simulink model "NDT_Localization"  (R2022a)
settings: Solver=FixedStepAuto  StartTime=0.0  StopTime=10.0  RelTol=1e-3
model workspace (MAT data in the model file):
  SL_ROS_VariableLengthArrays_MaxSizes : object (value not decoded)
undefined symbols (not defined in the file or in its folder): null
libraries: ros2lib x9, robotlib x8, simulink x1
(part 11 of 12)

== matlab function NDT_Localization/observation_callback/check_localizer/If Action Subsystem/register_measurement_impl/If Action Subsystem/If Action Subsystem/solve/If Action Subsystem1/For Iterator Subsystem/compute_next_step/If Action Subsystem1/For Iterator Subsystem/If Action Subsystem/If Action Subsystem3/If Action Subsystem/f_u/gradient_angle/ga_a ==
  data: x input; out output; y input; z input
function out = fcn(x, y, z)
out = zeros(1,3); 
out(1) = x;
out(2) = y;
out(3) = z;

== matlab function NDT_Localization/observation_callback/check_localizer/If Action Subsystem/register_measurement_impl/If Action Subsystem/If Action Subsystem/solve/If Action Subsystem1/For Iterator Subsystem/compute_next_step/If Action Subsystem1/For Iterator Subsystem/If Action Subsystem/If Action Subsystem3/If Action Subsystem/f_u/gradient_angle/ga_b ==
  data: x input; out output; y input; z input
function out = fcn(x, y, z)
out = zeros(1,3); 
out(1) = x;
out(2) = y;
out(3) = z;

== matlab function NDT_Localization/observation_callback/check_localizer/If Action Subsystem/register_measurement_impl/If Action Subsystem/If Action Subsystem/solve/If Action Subsystem1/For Iterator Subsystem/compute_next_step/If Action Subsystem1/For Iterator Subsystem/If Action Subsystem/If Action Subsystem3/If Action Subsystem/f_u/gradient_angle/ga_c ==
  data: x input; out output; y input; z input
function out = fcn(x, y, z)
out = zeros(1,3); 
out(1) = x;
out(2) = y;
out(3) = z;

== matlab function NDT_Localization/observation_callback/check_localizer/If Action Subsystem/register_measurement_impl/If Action Subsystem/If Action Subsystem/solve/If Action Subsystem1/For Iterator Subsystem/compute_next_step/If Action Subsystem1/For Iterator Subsystem/If Action Subsystem/If Action Subsystem3/If Action Subsystem/f_u/gradient_angle/ga_d ==
  data: x input; out output; y input; z input
function out = fcn(x, y, z)
out = zeros(1,3); 
out(1) = x;
out(2) = y;
out(3) = z;

== matlab function NDT_Localization/observation_callback/check_localizer/If Action Subsystem/register_measurement_impl/If Action Subsystem/If Action Subsystem/solve/If Action Subsystem1/For Iterator Subsystem/compute_next_step/If Action Subsystem1/For Iterator Subsystem/If Action Subsystem/If Action Subsystem3/If Action Subsystem/f_u/gradient_angle/ga_e ==
  data: x input; out output; y input; z input
function out = fcn(x, y, z)
out = zeros(1,3); 
out(1) = x;
out(2) = y;
out(3) = z;

== matlab function NDT_Localization/observation_callback/check_localizer/If Action Subsystem/register_measurement_impl/If Action Subsystem/If Action Subsystem/solve/If Action Subsystem1/For Iterator Subsystem/compute_next_step/If Action Subsystem1/For Iterator Subsystem/If Action Subsystem/If Action Subsystem3/If Action Subsystem/f_u/gradient_angle/ga_f ==
  data: x input; out output; y input; z input
function out = fcn(x, y, z)
out = zeros(1,3); 
out(1) = x;
out(2) = y;
out(3) = z;

== matlab function NDT_Localization/observation_callback/check_localizer/If Action Subsystem/register_measurement_impl/If Action Subsystem/If Action Subsystem/solve/If Action Subsystem1/For Iterator Subsystem/compute_next_step/If Action Subsystem1/For Iterator Subsystem/If Action Subsystem/If Action Subsystem3/If Action Subsystem/f_u/gradient_angle/ga_g ==
  data: x input; out output; y input; z input
function out = fcn(x, y, z)
out = zeros(1,3); 
out(1) = x;
out(2) = y;
out(3) = z;

== matlab function NDT_Localization/observation_callback/check_localizer/If Action Subsystem/register_measurement_impl/If Action Subsystem/If Action Subsystem/solve/If Action Subsystem1/For Iterator Subsystem/compute_next_step/If Action Subsystem1/For Iterator Subsystem/If Action Subsystem/If Action Subsystem3/If Action Subsystem/f_u/gradient_angle/ga_h ==
  data: x input; out output; y input; z input
function out = fcn(x, y, z)
out = zeros(1,3); 
out(1) = x;
out(2) = y;
out(3) = z;

== matlab function NDT_Localization/init//param/If Action Subsystem/set_jacobian ==
  data: jacobian output
function jacobian = fcn()

jacobian = zeros(6,1,"single");

== matlab function NDT_Localization/observation_callback/check_localizer/If Action Subsystem/register_measurement_impl/If Action Subsystem/If Action Subsystem/solve/If Action Subsystem1/For Iterator Subsystem/compute_next_step/If Action Subsystem1/For Iterator Subsystem/If Action Subsystem/If Action Subsystem3/If Action Subsystem/f_u/point_gradient ==
  data: hessian output; ga_a input; ga_b input; ga_c input; ga_d input; ga_e input; ga_f input; ga_g input; ga_h input
function hessian = fcn(ga_a, ga_b, ga_c, ga_d, ga_e, ga_f, ga_g, ga_h)

hessian = zeros(3,6,"single");
hessian(1,3) = ga_a;
hessian(2,3) = ga_b;
hessian(0,4) = ga_c;
hessian(1,4) = ga_d;
hessian(2,4) = ga_e;
hessian(0,5) = ga_f;
hessian(1,5) = ga_g;
hessian(2,5) = ga_h;

== matlab function NDT_Localization/observation_callback/check_localizer/If Action Subsystem/register_measurement_impl/If Action Subsystem/If Action Subsystem/solve/If Action Subsystem1/For Iterator Subsystem/compute_next_step/If Action Subsystem1/For Iterator Subsystem/If Action Subsystem/If Action Subsystem3/If Action Subsystem/f_u/set_jacobian ==
  data: jacobian output
function jacobian = fcn()

jacobian = zeros(6,1,"single");

== matlab function NDT_Localization/observation_callback/check_localizer/If Action Subsystem/register_measurement_impl/If Action Subsystem/If Action Subsystem/solve/If Action Subsystem1/For Iterator Subsystem/compute_next_step/If Action Subsystem1/f_l/initial_objective_function/For Iterator Subsystem/Affine ==
  data: out output; u input
function out = fcn(u)

tform = affine3d;
pt = pointCloud(u);
xyz = pctransform(pt,tform);
out = xyz.Location;

== matlab function NDT_Localization/observation_callback/check_localizer/If Action Subsystem/register_measurement_impl/If Action Subsystem/If Action Subsystem/solve/If Action Subsystem1/For Iterator Subsystem/compute_next_step/If Action Subsystem1/f_l/initial_objective_function/For Iterator Subsystem/MATLAB Function ==
  data: data input; pt output; index input
function pt = fcn(data,index)

pt = data(index);

== matlab function NDT_Localization/observation_callback/check_localizer/If Action Subsystem/register_measurement_impl/If Action Subsystem/If Action Subsystem/solve/If Action Subsystem1/For Iterator Subsystem/compute_next_step/If Action Subsystem1/f_l/initial_objective_function/For Iterator Subsystem/gradient_jaco/gradient_col ==
  data: index input; gradient input; y output
function y = fcn(index,gradient)

y = gradient(:,index);

== matlab function NDT_Localization/observation_callback/check_localizer/If Action Subsystem/register_measurement_impl/If Action Subsystem/If Action Subsystem/solve/If Action Subsystem1/For Iterator Subsystem/compute_next_step/If Action Subsystem1/f_l/initial_objective_function/For Iterator Subsystem/gradient_jaco/jaco_add ==
  data: jacobian input; jacobian output; index input; num input
function jacobian = fcn(jacobian,index,num)

jacobian(index) = jacobian(index)+num;

== matlab function NDT_Localization/observation_callback/check_localizer/If Action Subsystem/register_measurement_impl/If Action Subsystem/If Action Subsystem/solve/If Action Subsystem1/For Iterator Subsystem/compute_next_step/If Action Subsystem1/For Iterator Subsystem/If Action Subsystem/MATLAB Function ==
  data: a_t input; y output
function y = fcn(a_t)

y = isnan(a_t);

== matlab function NDT_Localization/observation_callback/check_localizer/If Action Subsystem/register_measurement_impl/If Action Subsystem/If Action Subsystem/solve/If Action Subsystem1/For Iterator Subsystem/compute_next_step/If Action Subsystem1/f_l/initial_objective_function/angle_params/MATLAB Function ==
  data: x output; u input; y output; z output
function [x,y,z] = fcn(u)
x = u(3);
y = u(4);
z = u(5);

== matlab function NDT_Localization/observation_callback/check_localizer/If Action Subsystem/register_measurement_impl/If Action Subsystem/If Action Subsystem/solve/If Action Subsystem1/For Iterator Subsystem/compute_next_step/If Action Subsystem1/f_l/initial_objective_function/gradient_angle/ga_a ==
  data: x input; out output; y input; z input
function out = fcn(x, y, z)
out = zeros(1,3); 
out(1) = x;
out(2) = y;
out(3) = z;

== matlab function NDT_Localization/observation_callback/check_localizer/If Action Subsystem/register_measurement_impl/If Action Subsystem/If Action Subsystem/solve/If Action Subsystem1/For Iterator Subsystem/compute_next_step/If Action Subsystem1/f_l/initial_objective_function/gradient_angle/ga_b ==
  data: x input; out output; y input; z input
function out = fcn(x, y, z)
out = zeros(1,3); 
out(1) = x;
out(2) = y;
out(3) = z;

== matlab function NDT_Localization/observation_callback/check_localizer/If Action Subsystem/register_measurement_impl/If Action Subsystem/If Action Subsystem/solve/If Action Subsystem1/For Iterator Subsystem/compute_next_step/If Action Subsystem1/f_l/initial_objective_function/gradient_angle/ga_c ==
  data: x input; out output; y input; z input
function out = fcn(x, y, z)
out = zeros(1,3); 
out(1) = x;
out(2) = y;
out(3) = z;

== matlab function NDT_Localization/observation_callback/check_localizer/If Action Subsystem/register_measurement_impl/If Action Subsystem/If Action Subsystem/solve/If Action Subsystem1/For Iterator Subsystem/compute_next_step/If Action Subsystem1/f_l/initial_objective_function/gradient_angle/ga_d ==
  data: x input; out output; y input; z input
function out = fcn(x, y, z)
out = zeros(1,3); 
out(1) = x;
out(2) = y;
out(3) = z;

== matlab function NDT_Localization/observation_callback/check_localizer/If Action Subsystem/register_measurement_impl/If Action Subsystem/If Action Subsystem/solve/If Action Subsystem1/For Iterator Subsystem/compute_next_step/If Action Subsystem1/f_l/initial_objective_function/gradient_angle/ga_e ==
  data: x input; out output; y input; z input
function out = fcn(x, y, z)
out = zeros(1,3); 
out(1) = x;
out(2) = y;
out(3) = z;

== matlab function NDT_Localization/observation_callback/check_localizer/If Action Subsystem/register_measurement_impl/If Action Subsystem/If Action Subsystem/solve/If Action Subsystem1/For Iterator Subsystem/compute_next_step/If Action Subsystem1/f_l/initial_objective_function/gradient_angle/ga_f ==
  data: x input; out output; y input; z input
function out = fcn(x, y, z)
out = zeros(1,3); 
out(1) = x;
out(2) = y;
out(3) = z;

== matlab function NDT_Localization/observation_callback/check_localizer/If Action Subsystem/register_measurement_impl/If Action Subsystem/If Action Subsystem/solve/If Action Subsystem1/For Iterator Subsystem/compute_next_step/If Action Subsystem1/f_l/initial_objective_function/gradient_angle/ga_g ==
  data: x input; out output; y input; z input
function out = fcn(x, y, z)
out = zeros(1,3); 
out(1) = x;
out(2) = y;
out(3) = z;

== matlab function NDT_Localization/observation_callback/check_localizer/If Action Subsystem/register_measurement_impl/If Action Subsystem/If Action Subsystem/solve/For Iterator Subsystem/MATLAB Function ==
  data: data input; pt output; index input
function pt = fcn(data,index)

pt = data(index);

== matlab function NDT_Localization/observation_callback/check_localizer/If Action Subsystem/register_measurement_impl/If Action Subsystem/If Action Subsystem/solve/If Action Subsystem1/For Iterator Subsystem/compute_next_step/If Action Subsystem1/f_l/initial_objective_function/gradient_angle/ga_h ==
  data: x input; out output; y input; z input
function out = fcn(x, y, z)
out = zeros(1,3); 
out(1) = x;
out(2) = y;
out(3) = z;

== matlab function NDT_Localization/observation_callback/check_localizer/If Action Subsystem/register_measurement_impl/If Action Subsystem/If Action Subsystem/solve/If Action Subsystem1/For Iterator Subsystem/compute_next_step/If Action Subsystem1/f_l/initial_objective_function/point_gradient ==
  data: hessian output; ga_a input; ga_b input; ga_c input; ga_d input; ga_e input; ga_f input; ga_g input; ga_h input
function hessian = fcn(ga_a, ga_b, ga_c, ga_d, ga_e, ga_f, ga_g, ga_h)

hessian = zeros(3,6,"single");
hessian(1,3) = ga_a;
hessian(2,3) = ga_b;
hessian(0,4) = ga_c;
hessian(1,4) = ga_d;
hessian(2,4) = ga_e;
hessian(0,5) = ga_f;
hessian(1,5) = ga_g;
hessian(2,5) = ga_h;

== matlab function NDT_Localization/observation_callback/check_localizer/If Action Subsystem/register_measurement_impl/If Action Subsystem/If Action Subsystem/solve/If Action Subsystem1/For Iterator Subsystem/compute_next_step/If Action Subsystem1/f_l/initial_objective_function/set_jacobian ==
  data: jacobian output
function jacobian = fcn()

jacobian = zeros(6,1,"single");

== matlab function NDT_Localization/observation_callback/check_localizer/If Action Subsystem/register_measurement_impl/If Action Subsystem/If Action Subsystem/solve/If Action Subsystem1/For Iterator Subsystem/compute_next_step/If Action Subsystem1/f_l/objective_function/For Iterator Subsystem/Affine ==
  data: out output; u input
function out = fcn(u)

tform = affine3d;
pt = pointCloud(u);
xyz = pctransform(pt,tform);
out = xyz.Location;

== matlab function NDT_Localization/observation_callback/check_localizer/If Action Subsystem/register_measurement_impl/If Action Subsystem/If Action Subsystem/solve/If Action Subsystem1/For Iterator Subsystem/compute_next_step/If Action Subsystem1/f_l/objective_function/For Iterator Subsystem/MATLAB Function ==
  data: data input; pt output; index input
function pt = fcn(data,index)

pt = data(index);

== matlab function NDT_Localization/observation_callback/check_localizer/If Action Subsystem/register_measurement_impl/If Action Subsystem/If Action Subsystem/solve/If Action Subsystem1/For Iterator Subsystem/compute_next_step/If Action Subsystem1/f_l/objective_function/For Iterator Subsystem/gradient_jaco/gradient_col ==
  data: index input; gradient input; y output
function y = fcn(index,gradient)

y = gradient(:,index);

== matlab function NDT_Localization/observation_callback/check_localizer/If Action Subsystem/register_measurement_impl/If Action Subsystem/If Action Subsystem/solve/If Action Subsystem1/For Iterator Subsystem/compute_next_step/If Action Subsystem1/f_l/objective_function/For Iterator Subsystem/gradient_jaco/jaco_add ==
  data: jacobian input; jacobian output; index input; num input
function jacobian = fcn(jacobian,index,num)

jacobian(index) = jacobian(index)+num;

== matlab function NDT_Localization/observation_callback/check_localizer/If Action Subsystem/register_measurement_impl/If Action Subsystem/If Action Subsystem/solve/If Action Subsystem1/For Iterator Subsystem/compute_next_step/If Action Subsystem1/f_l/objective_function/angle_params/MATLAB Function ==
  data: x output; u input; y output; z output
function [x,y,z] = fcn(u)
x = u(3);
y = u(4);
z = u(5);

== matlab function NDT_Localization/observation_callback/check_localizer/If Action Subsystem/register_measurement_impl/If Action Subsystem/If Action Subsystem/solve/If Action Subsystem1/For Iterator Subsystem/compute_next_step/If Action Subsystem1/f_l/objective_function/gradient_angle/ga_a ==
  data: x input; out output; y input; z input
function out = fcn(x, y, z)
out = zeros(1,3); 
out(1) = x;
out(2) = y;
out(3) = z;

== matlab function NDT_Localization/observation_callback/check_localizer/If Action Subsystem/register_measurement_impl/If Action Subsystem/If Action Subsystem/solve/For Iterator Subsystem/gradient_jaco/jaco_add ==
  data: jacobian input; jacobian output; index input; num input
function jacobian = fcn(jacobian,index,num)

jacobian(index) = jacobian(index)+num;

== matlab function NDT_Localization/observation_callback/check_localizer/If Action Subsystem/register_measurement_impl/If Action Subsystem/If Action Subsystem/solve/If Action Subsystem1/For Iterator Subsystem/compute_next_step/If Action Subsystem1/f_l/objective_function/gradient_angle/ga_b ==
  data: x input; out output; y input; z input
function out = fcn(x, y, z)
out = zeros(1,3); 
out(1) = x;
out(2) = y;
out(3) = z;

== matlab function NDT_Localization/observation_callback/check_localizer/If Action Subsystem/register_measurement_impl/If Action Subsystem/If Action Subsystem/solve/If Action Subsystem1/For Iterator Subsystem/compute_next_step/If Action Subsystem1/f_l/objective_function/gradient_angle/ga_c ==
  data: x input; out output; y input; z input
function out = fcn(x, y, z)
out = zeros(1,3); 
out(1) = x;
out(2) = y;
out(3) = z;

== matlab function NDT_Localization/observation_callback/check_localizer/If Action Subsystem/register_measurement_impl/If Action Subsystem/If Action Subsystem/solve/If Action Subsystem1/For Iterator Subsystem/compute_next_step/If Action Subsystem1/f_l/objective_function/gradient_angle/ga_d ==
  data: x input; out output; y input; z input
function out = fcn(x, y, z)
out = zeros(1,3); 
out(1) = x;
out(2) = y;
out(3) = z;

== matlab function NDT_Localization/observation_callback/check_localizer/If Action Subsystem/register_measurement_impl/If Action Subsystem/If Action Subsystem/solve/If Action Subsystem1/For Iterator Subsystem/compute_next_step/If Action Subsystem1/f_l/objective_function/gradient_angle/ga_e ==
  data: x input; out output; y input; z input
function out = fcn(x, y, z)
out = zeros(1,3); 
out(1) = x;
out(2) = y;
out(3) = z;

== matlab function NDT_Localization/observation_callback/check_localizer/If Action Subsystem/register_measurement_impl/If Action Subsystem/If Action Subsystem/solve/If Action Subsystem1/For Iterator Subsystem/compute_next_step/If Action Subsystem1/f_l/objective_function/gradient_angle/ga_f ==
  data: x input; out output; y input; z input
function out = fcn(x, y, z)
out = zeros(1,3); 
out(1) = x;
out(2) = y;
out(3) = z;

== matlab function NDT_Localization/observation_callback/check_localizer/If Action Subsystem/register_measurement_impl/If Action Subsystem/If Action Subsystem/solve/If Action Subsystem1/For Iterator Subsystem/compute_next_step/If Action Subsystem1/f_l/objective_function/gradient_angle/ga_g ==
  data: x input; out output; y input; z input
function out = fcn(x, y, z)
out = zeros(1,3); 
out(1) = x;
out(2) = y;
out(3) = z;

== matlab function NDT_Localization/observation_callback/check_localizer/If Action Subsystem/register_measurement_impl/If Action Subsystem/If Action Subsystem/solve/If Action Subsystem1/For Iterator Subsystem/compute_next_step/If Action Subsystem1/f_l/objective_function/gradient_angle/ga_h ==
  data: x input; out output; y input; z input
function out = fcn(x, y, z)
out = zeros(1,3); 
out(1) = x;
out(2) = y;
out(3) = z;

== matlab function NDT_Localization/observation_callback/check_localizer/If Action Subsystem/register_measurement_impl/If Action Subsystem/If Action Subsystem/solve/If Action Subsystem1/For Iterator Subsystem/compute_next_step/If Action Subsystem1/f_l/objective_function/point_gradient ==
  data: hessian output; ga_a input; ga_b input; ga_c input; ga_d input; ga_e input; ga_f input; ga_g input; ga_h input
function hessian = fcn(ga_a, ga_b, ga_c, ga_d, ga_e, ga_f, ga_g, ga_h)

hessian = zeros(3,6,"single");
hessian(1,3) = ga_a;
hessian(2,3) = ga_b;
hessian(0,4) = ga_c;
hessian(1,4) = ga_d;
hessian(2,4) = ga_e;
hessian(0,5) = ga_f;
hessian(1,5) = ga_g;
hessian(2,5) = ga_h;

== matlab function NDT_Localization/observation_callback/check_localizer/If Action Subsystem/register_measurement_impl/If Action Subsystem/If Action Subsystem/solve/If Action Subsystem1/For Iterator Subsystem/compute_next_step/If Action Subsystem1/f_l/objective_function/set_jacobian ==
  data: jacobian output
function jacobian = fcn()

jacobian = zeros(6,1,"single");

== matlab function NDT_Localization/observation_callback/check_localizer/If Action Subsystem/register_measurement_impl/If Action Subsystem/If Action Subsystem/solve/If Action Subsystem1/For Iterator Subsystem/compute_next_step/If Action Subsystem1/f_u/initial_objective_function/For Iterator Subsystem/Affine ==
  data: out output; u input
function out = fcn(u)

tform = affine3d;
pt = pointCloud(u);
xyz = pctransform(pt,tform);
out = xyz.Location;

== matlab function NDT_Localization/observation_callback/check_localizer/If Action Subsystem/register_measurement_impl/If Action Subsystem/If Action Subsystem/solve/For Iterator Subsystem/Affine ==
  data: out output; u input
function out = fcn(u)

tform = affine3d;
pt = pointCloud(u);
xyz = pctransform(pt,tform);
out = xyz.Location;

== matlab function NDT_Localization/observation_callback/check_localizer/If Action Subsystem/register_measurement_impl/If Action Subsystem/If Action Subsystem/solve/If Action Subsystem1/For Iterator Subsystem/compute_next_step/If Action Subsystem1/f_u/initial_objective_function/For Iterator Subsystem/MATLAB Function ==
  data: data input; pt output; index input
function pt = fcn(data,index)

pt = data(index);

== matlab function NDT_Localization/observation_callback/check_localizer/If Action Subsystem/register_measurement_impl/If Action Subsystem/If Action Subsystem/solve/If Action Subsystem1/For Iterator Subsystem/compute_next_step/If Action Subsystem1/f_u/initial_objective_function/For Iterator Subsystem/gradient_jaco/gradient_col ==
  data: index input; gradient input; y output
function y = fcn(index,gradient)

y = gradient(:,index);

== matlab function NDT_Localization/observation_callback/check_localizer/If Action Subsystem/register_measurement_impl/If Action Subsystem/If Action Subsystem/solve/If Action Subsystem1/For Iterator Subsystem/compute_next_step/If Action Subsystem1/f_u/initial_objective_function/For Iterator Subsystem/gradient_jaco/jaco_add ==
  data: jacobian input; jacobian output; index input; num input
function jacobian = fcn(jacobian,index,num)

jacobian(index) = jacobian(index)+num;

== matlab function NDT_Localization/observation_callback/check_localizer/If Action Subsystem/register_measurement_impl/If Action Subsystem/If Action Subsystem/solve/If Action Subsystem1/For Iterator Subsystem/compute_next_step/If Action Subsystem1/f_u/initial_objective_function/angle_params/MATLAB Function ==
  data: x output; u input; y output; z output
function [x,y,z] = fcn(u)
x = u(3);
y = u(4);
z = u(5);

== matlab function NDT_Localization/observation_callback/check_localizer/If Action Subsystem/register_measurement_impl/If Action Subsystem/If Action Subsystem/solve/If Action Subsystem1/For Iterator Subsystem/compute_next_step/If Action Subsystem1/f_u/initial_objective_function/gradient_angle/ga_a ==
  data: x input; out output; y input; z input
function out = fcn(x, y, z)
out = zeros(1,3); 
out(1) = x;
out(2) = y;
out(3) = z;

== matlab function NDT_Localization/observation_callback/check_localizer/If Action Subsystem/register_measurement_impl/If Action Subsystem/If Action Subsystem/solve/If Action Subsystem1/For Iterator Subsystem/compute_next_step/If Action Subsystem1/f_u/initial_objective_function/gradient_angle/ga_b ==
  data: x input; out output; y input; z input
function out = fcn(x, y, z)
out = zeros(1,3); 
out(1) = x;
out(2) = y;
out(3) = z;

== matlab function NDT_Localization/observation_callback/check_localizer/If Action Subsystem/register_measurement_impl/If Action Subsystem/If Action Subsystem/solve/If Action Subsystem1/For Iterator Subsystem/compute_next_step/If Action Subsystem1/f_u/initial_objective_function/gradient_angle/ga_c ==
  data: x input; out output; y input; z input
function out = fcn(x, y, z)
out = zeros(1,3); 
out(1) = x;
out(2) = y;
out(3) = z;

== matlab function NDT_Localization/observation_callback/check_localizer/If Action Subsystem/register_measurement_impl/If Action Subsystem/If Action Subsystem/solve/If Action Subsystem1/For Iterator Subsystem/compute_next_step/If Action Subsystem1/f_u/initial_objective_function/gradient_angle/ga_d ==
  data: x input; out output; y input; z input
function out = fcn(x, y, z)
out = zeros(1,3); 
out(1) = x;
out(2) = y;
out(3) = z;

== matlab function NDT_Localization/observation_callback/check_localizer/If Action Subsystem/register_measurement_impl/If Action Subsystem/If Action Subsystem/solve/point_gradient ==
  data: hessian output; ga_a input; ga_b input; ga_c input; ga_d input; ga_e input; ga_f input; ga_g input; ga_h input
function hessian = fcn(ga_a, ga_b, ga_c, ga_d, ga_e, ga_f, ga_g, ga_h)

hessian = zeros(3,6,"single");
hessian(1,3) = ga_a;
hessian(2,3) = ga_b;
hessian(0,4) = ga_c;
hessian(1,4) = ga_d;
hessian(2,4) = ga_e;
hessian(0,5) = ga_f;
hessian(1,5) = ga_g;
hessian(2,5) = ga_h;

== matlab function NDT_Localization/observation_callback/check_localizer/If Action Subsystem/register_measurement_impl/If Action Subsystem/If Action Subsystem/solve/If Action Subsystem1/For Iterator Subsystem/compute_next_step/If Action Subsystem1/f_u/initial_objective_function/gradient_angle/ga_e ==
  data: x input; out output; y input; z input
function out = fcn(x, y, z)
out = zeros(1,3); 
out(1) = x;
out(2) = y;
out(3) = z;

== matlab function NDT_Localization/observation_callback/check_localizer/If Action Subsystem/register_measurement_impl/If Action Subsystem/If Action Subsystem/solve/If Action Subsystem1/For Iterator Subsystem/compute_next_step/If Action Subsystem1/f_u/initial_objective_function/gradient_angle/ga_f ==
  data: x input; out output; y input; z input
function out = fcn(x, y, z)
out = zeros(1,3); 
out(1) = x;
out(2) = y;
out(3) = z;

== matlab function NDT_Localization/observation_callback/check_localizer/If Action Subsystem/register_measurement_impl/If Action Subsystem/If Action Subsystem/solve/If Action Subsystem1/For Iterator Subsystem/compute_next_step/If Action Subsystem1/f_u/initial_objective_function/gradient_angle/ga_g ==
  data: x input; out output; y input; z input
function out = fcn(x, y, z)
out = zeros(1,3); 
out(1) = x;
out(2) = y;
out(3) = z;

== matlab function NDT_Localization/observation_callback/check_localizer/If Action Subsystem/register_measurement_impl/If Action Subsystem/If Action Subsystem/solve/If Action Subsystem1/For Iterator Subsystem/compute_next_step/If Action Subsystem1/f_u/initial_objective_function/gradient_angle/ga_h ==
  data: x input; out output; y input; z input
function out = fcn(x, y, z)
out = zeros(1,3); 
out(1) = x;
out(2) = y;
out(3) = z;

== matlab function NDT_Localization/observation_callback/check_localizer/If Action Subsystem/register_measurement_impl/If Action Subsystem/If Action Subsystem/solve/If Action Subsystem1/For Iterator Subsystem/compute_next_step/If Action Subsystem1/f_u/initial_objective_function/point_gradient ==
  data: hessian output; ga_a input; ga_b input; ga_c input; ga_d input; ga_e input; ga_f input; ga_g input; ga_h input
function hessian = fcn(ga_a, ga_b, ga_c, ga_d, ga_e, ga_f, ga_g, ga_h)

hessian = zeros(3,6,"single");
hessian(1,3) = ga_a;
hessian(2,3) = ga_b;
hessian(0,4) = ga_c;
hessian(1,4) = ga_d;
hessian(2,4) = ga_e;
hessian(0,5) = ga_f;
hessian(1,5) = ga_g;
hessian(2,5) = ga_h;

== matlab function NDT_Localization/observation_callback/check_localizer/If Action Subsystem/register_measurement_impl/If Action Subsystem/If Action Subsystem/solve/If Action Subsystem1/For Iterator Subsystem/compute_next_step/If Action Subsystem1/f_u/initial_objective_function/set_jacobian ==
  data: jacobian output
function jacobian = fcn()

jacobian = zeros(6,1,"single");

== matlab function NDT_Localization/observation_callback/check_localizer/If Action Subsystem/register_measurement_impl/If Action Subsystem/If Action Subsystem/solve/If Action Subsystem1/For Iterator Subsystem/compute_next_step/If Action Subsystem1/f_u/objective_function/For Iterator Subsystem/Affine ==
  data: out output; u input
function out = fcn(u)

tform = affine3d;
pt = pointCloud(u);
xyz = pctransform(pt,tform);
out = xyz.Location;

== matlab function NDT_Localization/observation_callback/check_localizer/If Action Subsystem/register_measurement_impl/If Action Subsystem/If Action Subsystem/solve/If Action Subsystem1/For Iterator Subsystem/compute_next_step/If Action Subsystem1/f_u/objective_function/For Iterator Subsystem/MATLAB Function ==
  data: data input; pt output; index input
function pt = fcn(data,index)

pt = data(index);

== matlab function NDT_Localization/observation_callback/check_localizer/If Action Subsystem/register_measurement_impl/If Action Subsystem/If Action Subsystem/solve/If Action Subsystem1/For Iterator Subsystem/compute_next_step/If Action Subsystem1/f_u/objective_function/For Iterator Subsystem/gradient_jaco/gradient_col ==
  data: index input; gradient input; y output
function y = fcn(index,gradient)

y = gradient(:,index);

== matlab function NDT_Localization/observation_callback/check_localizer/If Action Subsystem/register_measurement_impl/If Action Subsystem/If Action Subsystem/solve/If Action Subsystem1/For Iterator Subsystem/compute_next_step/If Action Subsystem1/f_u/objective_function/For Iterator Subsystem/gradient_jaco/jaco_add ==
  data: jacobian input; jacobian output; index input; num input
function jacobian = fcn(jacobian,index,num)

jacobian(index) = jacobian(index)+num;

== matlab function NDT_Localization/observation_callback/check_localizer/If Action Subsystem/register_measurement_impl/If Action Subsystem/If Action Subsystem/solve/If Action Subsystem1/For Iterator Subsystem/compute_next_step/If Action Subsystem1/f_u/objective_function/angle_params/MATLAB Function ==
  data: x output; u input; y output; z output
function [x,y,z] = fcn(u)
x = u(3);
y = u(4);
z = u(5);

== matlab function NDT_Localization/observation_callback/check_localizer/If Action Subsystem/register_measurement_impl/If Action Subsystem/If Action Subsystem/solve/If Action Subsystem1/For Iterator Subsystem/compute_next_step/If Action Subsystem1/f_u/objective_function/gradient_angle/ga_a ==
  data: x input; out output; y input; z input
function out = fcn(x, y, z)
out = zeros(1,3); 
out(1) = x;
out(2) = y;
out(3) = z;

== matlab function NDT_Localization/observation_callback/check_localizer/If Action Subsystem/register_measurement_impl/If Action Subsystem/If Action Subsystem/solve/If Action Subsystem1/For Iterator Subsystem/compute_next_step/If Action Subsystem1/f_u/objective_function/gradient_angle/ga_b ==
  data: x input; out output; y input; z input
function out = fcn(x, y, z)
out = zeros(1,3); 
out(1) = x;
out(2) = y;
out(3) = z;

== matlab function NDT_Localization/observation_callback/check_localizer/If Action Subsystem/register_measurement_impl/If Action Subsystem/If Action Subsystem/solve/If Action Subsystem1/For Iterator Subsystem/compute_next_step/If Action Subsystem1/f_u/objective_function/gradient_angle/ga_c ==
  data: x input; out output; y input; z input
function out = fcn(x, y, z)
out = zeros(1,3); 
out(1) = x;
out(2) = y;
out(3) = z;

== matlab function NDT_Localization/observation_callback/check_localizer/If Action Subsystem/register_measurement_impl/If Action Subsystem/If Action Subsystem/solve/If Action Subsystem1/For Iterator Subsystem/compute_next_step/If Action Subsystem1/f_u/objective_function/gradient_angle/ga_d ==
  data: x input; out output; y input; z input
function out = fcn(x, y, z)
out = zeros(1,3); 
out(1) = x;
out(2) = y;
out(3) = z;

== matlab function NDT_Localization/observation_callback/check_localizer/If Action Subsystem/register_measurement_impl/If Action Subsystem/If Action Subsystem/solve/If Action Subsystem1/For Iterator Subsystem/compute_next_step/If Action Subsystem1/f_u/objective_function/gradient_angle/ga_e ==
  data: x input; out output; y input; z input
function out = fcn(x, y, z)
out = zeros(1,3); 
out(1) = x;
out(2) = y;
out(3) = z;

== matlab function NDT_Localization/observation_callback/check_localizer/If Action Subsystem/register_measurement_impl/If Action Subsystem/If Action Subsystem/solve/For Iterator Subsystem/gradient_jaco/gradient_col ==
  data: index input; gradient input; y output
function y = fcn(index,gradient)

y = gradient(:,index);

== matlab function NDT_Localization/observation_callback/check_localizer/If Action Subsystem/register_measurement_impl/If Action Subsystem/If Action Subsystem/solve/If Action Subsystem1/For Iterator Subsystem/compute_next_step/If Action Subsystem1/f_u/objective_function/gradient_angle/ga_f ==
  data: x input; out output; y input; z input
function out = fcn(x, y, z)
out = zeros(1,3); 
out(1) = x;
out(2) = y;
out(3) = z;

== matlab function NDT_Localization/observation_callback/check_localizer/If Action Subsystem/register_measurement_impl/If Action Subsystem/If Action Subsystem/solve/If Action Subsystem1/For Iterator Subsystem/compute_next_step/If Action Subsystem1/f_u/objective_function/gradient_angle/ga_g ==
  data: x input; out output; y input; z input
function out = fcn(x, y, z)
out = zeros(1,3); 
out(1) = x;
out(2) = y;
out(3) = z;

== matlab function NDT_Localization/observation_callback/check_localizer/If Action Subsystem/register_measurement_impl/If Action Subsystem/If Action Subsystem/solve/If Action Subsystem1/For Iterator Subsystem/compute_next_step/If Action Subsystem1/f_u/objective_function/gradient_angle/ga_h ==
  data: x input; out output; y input; z input
function out = fcn(x, y, z)
out = zeros(1,3); 
out(1) = x;
out(2) = y;
out(3) = z;

== matlab function NDT_Localization/observation_callback/check_localizer/If Action Subsystem/register_measurement_impl/If Action Subsystem/If Action Subsystem/solve/If Action Subsystem1/For Iterator Subsystem/compute_next_step/If Action Subsystem1/f_u/objective_function/point_gradient ==
  data: hessian output; ga_a input; ga_b input; ga_c input; ga_d input; ga_e input; ga_f input; ga_g input; ga_h input
function hessian = fcn(ga_a, ga_b, ga_c, ga_d, ga_e, ga_f, ga_g, ga_h)

hessian = zeros(3,6,"single");
hessian(1,3) = ga_a;
hessian(2,3) = ga_b;
hessian(0,4) = ga_c;
hessian(1,4) = ga_d;
hessian(2,4) = ga_e;
hessian(0,5) = ga_f;
hessian(1,5) = ga_g;
hessian(2,5) = ga_h;

== matlab function NDT_Localization/observation_callback/check_localizer/If Action Subsystem/register_measurement_impl/If Action Subsystem/If Action Subsystem/solve/If Action Subsystem1/For Iterator Subsystem/compute_next_step/If Action Subsystem1/f_u/objective_function/set_jacobian ==
  data: jacobian output
function jacobian = fcn()

jacobian = zeros(6,1,"single");

== matlab function NDT_Localization/observation_callback/check_localizer/If Action Subsystem/register_measurement_impl/If Action Subsystem/If Action Subsystem/solve/If Action Subsystem1/For Iterator Subsystem/compute_next_step/If Action Subsystem1/phi_0/For Iterator Subsystem/Affine ==
  data: out output; u input
function out = fcn(u)

tform = affine3d;
pt = pointCloud(u);
xyz = pctransform(pt,tform);
out = xyz.Location;

== matlab function NDT_Localization/observation_callback/check_localizer/If Action Subsystem/register_measurement_impl/If Action Subsystem/If Action Subsystem/solve/If Action Subsystem1/For Iterator Subsystem/compute_next_step/If Action Subsystem1/phi_0/For Iterator Subsystem/MATLAB Function ==
  data: data input; pt output; index input
function pt = fcn(data,index)

pt = data(index);

== matlab function NDT_Localization/observation_callback/check_localizer/If Action Subsystem/register_measurement_impl/If Action Subsystem/If Action Subsystem/solve/If Action Subsystem1/For Iterator Subsystem/compute_next_step/If Action Subsystem1/phi_0/For Iterator Subsystem/gradient_jaco/gradient_col ==
  data: index input; gradient input; y output
function y = fcn(index,gradient)

y = gradient(:,index);

== matlab function NDT_Localization/observation_callback/check_localizer/If Action Subsystem/register_measurement_impl/If Action Subsystem/If Action Subsystem/solve/If Action Subsystem1/For Iterator Subsystem/compute_next_step/If Action Subsystem1/phi_0/For Iterator Subsystem/gradient_jaco/jaco_add ==
  data: jacobian input; jacobian output; index input; num input
function jacobian = fcn(jacobian,index,num)

jacobian(index) = jacobian(index)+num;

== matlab function NDT_Localization/observation_callback/check_localizer/If Action Subsystem/register_measurement_impl/If Action Subsystem/If Action Subsystem/solve/For Iterator Subsystem/For Iterator Subsystem/gradient_col_i ==
  data: index_i input; gradient input; y output
function y = fcn(index_i,gradient)

y = gradient(:,index_i);

== matlab function NDT_Localization/observation_callback/check_localizer/If Action Subsystem/register_measurement_impl/If Action Subsystem/If Action Subsystem/solve/If Action Subsystem1/For Iterator Subsystem/compute_next_step/If Action Subsystem1/phi_0/angle_params/MATLAB Function ==
  data: x output; u input; y output; z output
function [x,y,z] = fcn(u)
x = u(3);
y = u(4);
z = u(5);

== matlab function NDT_Localization/observation_callback/check_localizer/If Action Subsystem/register_measurement_impl/If Action Subsystem/If Action Subsystem/solve/If Action Subsystem1/For Iterator Subsystem/compute_next_step/If Action Subsystem1/phi_0/gradient_angle/ga_a ==
  data: x input; out output; y input; z input
function out = fcn(x, y, z)
out = zeros(1,3); 
out(1) = x;
out(2) = y;
out(3) = z;

== matlab function NDT_Localization/observation_callback/check_localizer/If Action Subsystem/register_measurement_impl/If Action Subsystem/If Action Subsystem/solve/If Action Subsystem1/For Iterator Subsystem/compute_next_step/If Action Subsystem1/phi_0/gradient_angle/ga_b ==
  data: x input; out output; y input; z input
function out = fcn(x, y, z)
out = zeros(1,3); 
out(1) = x;
out(2) = y;
out(3) = z;

== matlab function NDT_Localization/observation_callback/check_localizer/If Action Subsystem/register_measurement_impl/If Action Subsystem/If Action Subsystem/solve/If Action Subsystem1/For Iterator Subsystem/compute_next_step/If Action Subsystem1/phi_0/gradient_angle/ga_c ==
  data: x input; out output; y input; z input
function out = fcn(x, y, z)
out = zeros(1,3); 
out(1) = x;
out(2) = y;
out(3) = z;

== matlab function NDT_Localization/observation_callback/check_localizer/If Action Subsystem/register_measurement_impl/If Action Subsystem/If Action Subsystem/solve/If Action Subsystem1/For Iterator Subsystem/compute_next_step/If Action Subsystem1/phi_0/gradient_angle/ga_d ==
  data: x input; out output; y input; z input
function out = fcn(x, y, z)
out = zeros(1,3); 
out(1) = x;
out(2) = y;
out(3) = z;

== matlab function NDT_Localization/observation_callback/check_localizer/If Action Subsystem/register_measurement_impl/If Action Subsystem/If Action Subsystem/solve/If Action Subsystem1/For Iterator Subsystem/compute_next_step/If Action Subsystem1/phi_0/gradient_angle/ga_e ==
  data: x input; out output; y input; z input
function out = fcn(x, y, z)
out = zeros(1,3); 
out(1) = x;
out(2) = y;
out(3) = z;

== matlab function NDT_Localization/observation_callback/check_localizer/If Action Subsystem/register_measurement_impl/If Action Subsystem/If Action Subsystem/solve/If Action Subsystem1/For Iterator Subsystem/compute_next_step/If Action Subsystem1/phi_0/gradient_angle/ga_f ==
  data: x input; out output; y input; z input
function out = fcn(x, y, z)
out = zeros(1,3); 
out(1) = x;
out(2) = y;
out(3) = z;

== matlab function NDT_Localization/observation_callback/check_localizer/If Action Subsystem/register_measurement_impl/If Action Subsystem/If Action Subsystem/solve/If Action Subsystem1/For Iterator Subsystem/compute_next_step/If Action Subsystem1/phi_0/gradient_angle/ga_g ==
  data: x input; out output; y input; z input
function out = fcn(x, y, z)
out = zeros(1,3); 
out(1) = x;
out(2) = y;
out(3) = z;

== matlab function NDT_Localization/observation_callback/check_localizer/If Action Subsystem/register_measurement_impl/If Action Subsystem/If Action Subsystem/solve/If Action Subsystem1/For Iterator Subsystem/compute_next_step/If Action Subsystem1/phi_0/gradient_angle/ga_h ==
  data: x input; out output; y input; z input
function out = fcn(x, y, z)
out = zeros(1,3); 
out(1) = x;
out(2) = y;
out(3) = z;

== matlab function NDT_Localization/observation_callback/check_localizer/If Action Subsystem/register_measurement_impl/If Action Subsystem/If Action Subsystem/solve/For Iterator Subsystem/For Iterator Subsystem/hessian_add ==
  data: hessian input; hessian output; index_i input; index_j input; num input
function hessian = fcn(hessian,index_i,index_j,num)

hessian(index_i,index_j) = hessian(index_i,index_j)+num;

== matlab function NDT_Localization/observation_callback/check_localizer/If Action Subsystem/register_measurement_impl/If Action Subsystem/If Action Subsystem/solve/If Action Subsystem1/For Iterator Subsystem/compute_next_step/If Action Subsystem1/phi_0/point_gradient ==
  data: hessian output; ga_a input; ga_b input; ga_c input; ga_d input; ga_e input; ga_f input; ga_g input; ga_h input
function hessian = fcn(ga_a, ga_b, ga_c, ga_d, ga_e, ga_f, ga_g, ga_h)

hessian = zeros(3,6,"single");
hessian(1,3) = ga_a;
hessian(2,3) = ga_b;
hessian(0,4) = ga_c;
hessian(1,4) = ga_d;
hessian(2,4) = ga_e;
hessian(0,5) = ga_f;
hessian(1,5) = ga_g;
hessian(2,5) = ga_h;

== matlab function NDT_Localization/observation_callback/check_localizer/If Action Subsystem/register_measurement_impl/If Action Subsystem/If Action Subsystem/solve/If Action Subsystem1/For Iterator Subsystem/compute_next_step/If Action Subsystem1/phi_0/set_jacobian ==
  data: jacobian output
function jacobian = fcn()

jacobian = zeros(6,1,"single");

== matlab function NDT_Localization/observation_callback/check_localizer/If Action Subsystem/register_measurement_impl/If Action Subsystem/If Action Subsystem/solve/If Action Subsystem1/For Iterator Subsystem/compute_next_step/If Action Subsystem1/phi_t/For Iterator Subsystem/Affine ==
  data: out output; u input
function out = fcn(u)

tform = affine3d;
pt = pointCloud(u);
xyz = pctransform(pt,tform);
out = xyz.Location;

== matlab function NDT_Localization/observation_callback/check_localizer/If Action Subsystem/register_measurement_impl/If Action Subsystem/If Action Subsystem/solve/If Action Subsystem1/For Iterator Subsystem/compute_next_step/If Action Subsystem1/phi_t/For Iterator Subsystem/MATLAB Function ==
  data: data input; pt output; index input
function pt = fcn(data,index)

pt = data(index);

== matlab function NDT_Localization/observation_callback/check_localizer/If Action Subsystem/register_measurement_impl/If Action Subsystem/If Action Subsystem/solve/If Action Subsystem1/For Iterator Subsystem/compute_next_step/If Action Subsystem1/phi_t/For Iterator Subsystem/gradient_jaco/gradient_col ==
  data: index input; gradient input; y output
function y = fcn(index,gradient)

y = gradient(:,index);

== matlab function NDT_Localization/observation_callback/check_localizer/If Action Subsystem/register_measurement_impl/If Action Subsystem/If Action Subsystem/solve/If Action Subsystem1/For Iterator Subsystem/compute_next_step/If Action Subsystem1/phi_t/For Iterator Subsystem/gradient_jaco/jaco_add ==
  data: jacobian input; jacobian output; index input; num input
function jacobian = fcn(jacobian,index,num)

jacobian(index) = jacobian(index)+num;

== matlab function NDT_Localization/observation_callback/check_localizer/If Action Subsystem/register_measurement_impl/If Action Subsystem/If Action Subsystem/solve/If Action Subsystem1/For Iterator Subsystem/compute_next_step/If Action Subsystem1/phi_t/angle_params/MATLAB Function ==
  data: x output; u input; y output; z output
function [x,y,z] = fcn(u)
x = u(3);
y = u(4);
z = u(5);

== matlab function NDT_Localization/observation_callback/check_localizer/If Action Subsystem/register_measurement_impl/If Action Subsystem/If Action Subsystem/solve/If Action Subsystem1/For Iterator Subsystem/compute_next_step/If Action Subsystem1/phi_t/gradient_angle/ga_a ==
  data: x input; out output; y input; z input
function out = fcn(x, y, z)
out = zeros(1,3); 
out(1) = x;
out(2) = y;
out(3) = z;

== matlab function NDT_Localization/observation_callback/check_localizer/If Action Subsystem/register_measurement_impl/If Action Subsystem/If Action Subsystem/solve/If Action Subsystem1/For Iterator Subsystem/compute_next_step/If Action Subsystem1/phi_t/gradient_angle/ga_b ==
  data: x input; out output; y input; z input
function out = fcn(x, y, z)
out = zeros(1,3); 
out(1) = x;
out(2) = y;
out(3) = z;

== matlab function NDT_Localization/observation_callback/check_localizer/If Action Subsystem/register_measurement_impl/If Action Subsystem/If Action Subsystem/solve/If Action Subsystem1/For Iterator Subsystem/compute_next_step/If Action Subsystem1/phi_t/gradient_angle/ga_c ==
  data: x input; out output; y input; z input
function out = fcn(x, y, z)
out = zeros(1,3); 
out(1) = x;
out(2) = y;
out(3) = z;

== matlab function NDT_Localization/observation_callback/check_localizer/If Action Subsystem/register_measurement_impl/If Action Subsystem/If Action Subsystem/solve/If Action Subsystem1/For Iterator Subsystem/compute_next_step/If Action Subsystem1/phi_t/gradient_angle/ga_d ==
  data: x input; out output; y input; z input
function out = fcn(x, y, z)
out = zeros(1,3); 
out(1) = x;
out(2) = y;
out(3) = z;

== matlab function NDT_Localization/observation_callback/check_localizer/If Action Subsystem/register_measurement_impl/If Action Subsystem/If Action Subsystem/solve/For Iterator Subsystem/For Iterator Subsystem/MATLAB Function ==
  data: u input; y output
function y = fcn(u)

y = size(u,2);

== matlab function NDT_Localization/observation_callback/check_localizer/If Action Subsystem/register_measurement_impl/If Action Subsystem/If Action Subsystem/solve/If Action Subsystem1/For Iterator Subsystem/compute_next_step/If Action Subsystem1/phi_t/gradient_angle/ga_e ==
  data: x input; out output; y input; z input
function out = fcn(x, y, z)
out = zeros(1,3); 
out(1) = x;
out(2) = y;
out(3) = z;

== matlab function NDT_Localization/observation_callback/check_localizer/If Action Subsystem/register_measurement_impl/If Action Subsystem/If Action Subsystem/solve/If Action Subsystem1/For Iterator Subsystem/compute_next_step/If Action Subsystem1/phi_t/gradient_angle/ga_f ==
  data: x input; out output; y input; z input
function out = fcn(x, y, z)
out = zeros(1,3); 
out(1) = x;
out(2) = y;
out(3) = z;

== matlab function NDT_Localization/observation_callback/check_localizer/If Action Subsystem/register_measurement_impl/If Action Subsystem/If Action Subsystem/solve/If Action Subsystem1/For Iterator Subsystem/compute_next_step/If Action Subsystem1/phi_t/gradient_angle/ga_g ==
  data: x input; out output; y input; z input
function out = fcn(x, y, z)
out = zeros(1,3); 
out(1) = x;
out(2) = y;
out(3) = z;

== matlab function NDT_Localization/observation_callback/check_localizer/If Action Subsystem/register_measurement_impl/If Action Subsystem/If Action Subsystem/solve/If Action Subsystem1/For Iterator Subsystem/compute_next_step/If Action Subsystem1/phi_t/gradient_angle/ga_h ==
  data: x input; out output; y input; z input
function out = fcn(x, y, z)
out = zeros(1,3); 
out(1) = x;
out(2) = y;
out(3) = z;

== matlab function NDT_Localization/observation_callback/check_localizer/If Action Subsystem/register_measurement_impl/If Action Subsystem/If Action Subsystem/solve/If Action Subsystem1/For Iterator Subsystem/compute_next_step/If Action Subsystem1/phi_t/point_gradient ==
  data: hessian output; ga_a input; ga_b input; ga_c input; ga_d input; ga_e input; ga_f input; ga_g input; ga_h input
function hessian = fcn(ga_a, ga_b, ga_c, ga_d, ga_e, ga_f, ga_g, ga_h)

hessian = zeros(3,6,"single");
hessian(1,3) = ga_a;
hessian(2,3) = ga_b;
hessian(0,4) = ga_c;
hessian(1,4) = ga_d;
hessian(2,4) = ga_e;
hessian(0,5) = ga_f;
hessian(1,5) = ga_g;
hessian(2,5) = ga_h;

== matlab function NDT_Localization/map_callback/check_localizer/set_map/set_map_impl/insert/insert_/validate_pcl_map/check_fields/check_fields_name/For Iterator Subsystem/MATLAB Function ==
  data: data input string; index input; name input string; offset input; data1 input; data output; data1 output
function [data,data1] = fcn(data,index, name, offset,data1)
data(index)=name;
data1(index)=offset;

== matlab function NDT_Localization/observation_callback/check_localizer/If Action Subsystem/register_measurement_impl/If Action Subsystem/If Action Subsystem/solve/If Action Subsystem1/For Iterator Subsystem/compute_next_step/If Action Subsystem1/phi_t/set_jacobian ==
  data: jacobian output
function jacobian = fcn()

jacobian = zeros(6,1,"single");

== matlab function NDT_Localization/observation_callback/check_localizer/If Action Subsystem/register_measurement_impl/If Action Subsystem/If Action Subsystem/solve/If Action Subsystem1/For Iterator Subsystem/compute_next_step/If Action Subsystem1/psi_t/initial_objective_function/For Iterator Subsystem/Affine ==
  data: out output; u input
function out = fcn(u)

tform = affine3d;
pt = pointCloud(u);
xyz = pctransform(pt,tform);
out = xyz.Location;

== matlab function NDT_Localization/observation_callback/check_localizer/If Action Subsystem/register_measurement_impl/If Action Subsystem/If Action Subsystem/solve/If Action Subsystem1/For Iterator Subsystem/compute_next_step/If Action Subsystem1/psi_t/initial_objective_function/For Iterator Subsystem/MATLAB Function ==
  data: data input; pt output; index input
function pt = fcn(data,index)

pt = data(index);

== matlab function NDT_Localization/observation_callback/check_localizer/If Action Subsystem/register_measurement_impl/If Action Subsystem/If Action Subsystem/solve/For Iterator Subsystem/For Iterator Subsystem/gradient_col_j ==
  data: index_j input; gradient input; y output
function y = fcn(index_j,gradient)

y = gradient(:,index_j);
